simulink model "MADA3"  (R2020a)
settings: Solver=ode4  StartTime=start_time  StopTime=stop_time  FixedStep=fixed_step_size  MaxStep=1e-4  RelTol=1e-3
undefined symbols (not defined in the file): J, Ki, Kp, Lr, Ls, M, p, Rr, Rs, T_23, T_32
settings Model: Creator=deric  LastModifiedBy=deric

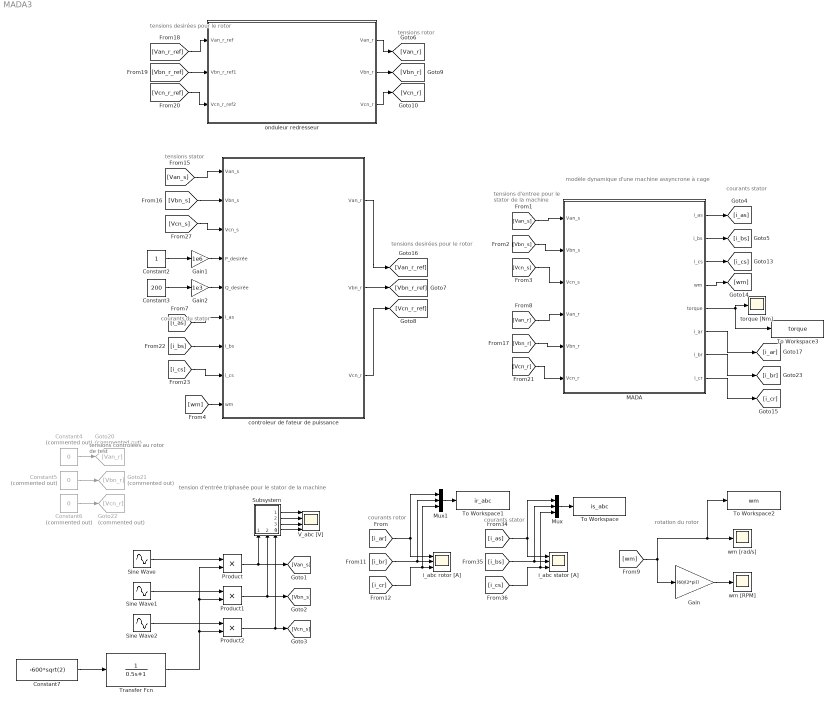
== system MADA3 ==
  note: tensions desirées
      | pour le rotor
  note: courants stator
  note: courants rotor
  note: tensions stator
  note: rotation du rotor
  note: tensions rotor
  note: tensions desirées
      | pour le rotor
  note: tensions controlées
      | au rotor de test
  note: tensions d'entree pour
      | le stator de la machine
  note: modèle dynamique d'une machine assyncrone à cage
  note: courants stator
  note: tension d'entrée triphasée pour le stator de la machine
  note: courants du stator
  Constant2 : Constant
  Constant3 : Constant  Value=200
  Constant4 : Constant  Commented=on  Value=0
  Constant5 : Constant  Commented=on  Value=0
  Constant6 : Constant  Commented=on  Value=0
  Constant7 : Constant  Value=-600*sqrt(2)
  Gain : Gain  Gain=(60/(2*pi))
  Gain1 : Gain  Gain=1e6
  Gain2 : Gain  Gain=1e3
  Goto20 : Goto  Commented=on  GotoTag=Van_r
  Goto21 : Goto  Commented=on  GotoTag=Vbn_r
  Goto22 : Goto  Commented=on  GotoTag=Vcn_r
  MADA : Subsystem
  Mux : Mux  Inputs=3
  Mux1 : Mux  Inputs=3
  Product : Product
  Product1 : Product
  Product2 : Product
  Sine Wave : Sin  Frequency=50*2*pi  SampleTime=0
  Sine Wave1 : Sin  Frequency=50*2*pi  Phase=-2*pi/3  SampleTime=0
  Sine Wave2 : Sin  Frequency=50*2*pi  Phase=(2*pi)/3  SampleTime=0
  Subsystem : Subsystem
      settings: PortSchema="{\"entries\":[{\"content\":{\"sides\":[{\"content\":{\"connectorIds\":[]},\"type\":\"ConnectorPlacement.EquallySpacedRectSide\",\"uuid\":\"f85b66a8-0283-4540-940c-33deb3ca5510\"},{\"content\":{\"connectorIds\":[\"Out1\",\"Out2\",\"Out3\",\"Out4\"],\"side\":\"RIGHT\"},\"type\":\"ConnectorPlacement.EquallySpacedRectSide\",\"uuid\":\"e99f7d2c-d092-4cab-bef3-1d0691980dab\"},{\"content\":{\"connectorIds\":[],\"side\":\"TOP\"},\"type\":\"ConnectorPlacement.EquallySpacedRectSide\",\"uuid\":\"dc5a25e5-8be2-48e2-ba29-fa1fa10bdc19\"},{\"content\":{\"connectorIds\":[\"In1\",\"In2\",\"In3\"],\"side\":\"BOTTOM\"},\"type\":\"ConnectorPlacement.EquallySpacedRectSide\",\"uuid\":\"6c390d1e-5fa5-44b0-aac6-b431b338384d\"}]},\"type\":\"ConnectorPlacement.EquallySpacedConnector\",\"uuid\":\"6ae22648-050b-430b-93b5-6047f057b4ba\"}],\"packageUris\":[\"http://schema.mathworks.com/mf0/Connector/19700101\"],\"version\":\"1.0\"}"
  To Workspace : ToWorkspace  VariableName=is_abc  SampleTime=-1
  To Workspace1 : ToWorkspace  VariableName=ir_abc  SampleTime=-1
  To Workspace2 : ToWorkspace  VariableName=wm  SampleTime=-1
  To Workspace3 : ToWorkspace  VariableName=torque  SampleTime=-1
  Transfer Fcn : TransferFcn  Denominator=[0.5 1]
  V_abc [V] : Scope  NumInputPorts=4
  controleur de fateur de puissance : Subsystem
  i_abc rotor [A] : Scope  NumInputPorts=3
  i_abc stator [A] : Scope  NumInputPorts=3
  onduleur redresseur : Subsystem
  torque [Nm] : Scope
  wm [RPM] : Scope
  wm [rad/s] : Scope
  wires:
  [wm] -> To Workspace2/1, wm [rad/s]/1, Gain/1
  Gain/1 -> wm [RPM]/1
  [Van_r_ref] -> onduleur redresseur/1(Van_r_ref)
  [Vbn_r_ref] -> onduleur redresseur/2(Vbn_r_ref1)
  [Vcn_r_ref] -> onduleur redresseur/3(Vcn_r_ref2)
  onduleur redresseur/1(Van_r) -> [Van_r]
  onduleur redresseur/2(Vbn_r) -> [Vbn_r]
  onduleur redresseur/3(Vcn_r) -> [Vcn_r]
  [i_ar] -> i_abc rotor [A]/1, Mux1/1
  [i_br] -> Mux1/2, i_abc rotor [A]/2
  [i_cr] -> Mux1/3, i_abc rotor [A]/3
  [i_cs] -> Mux/3, i_abc stator [A]/3
  [i_as] -> Mux/1, i_abc stator [A]/1
  [i_bs] -> Mux/2, i_abc stator [A]/2
  Mux/1 -> To Workspace/1
  Mux1/1 -> To Workspace1/1
  MADA/3(i_cs) -> [i_cs]
  MADA/4(wm) -> [wm]
  [Vcn_s] -> MADA/3(Vcn_s)
  [Van_s] -> MADA/1(Van_s)
  MADA/5(torque) -> To Workspace3/1, torque [Nm]/1
  [Vbn_s] -> MADA/2(Vbn_s)
  MADA/1(i_as) -> [i_as]
  MADA/2(i_bs) -> [i_bs]
  Subsystem/3(Out3) -> V_abc [V]/3
  Subsystem/2(Out2) -> V_abc [V]/2
  Subsystem/1(Out1) -> V_abc [V]/1
  Subsystem/4(Out4) -> V_abc [V]/4
  [Van_r] -> MADA/4(Van_r)
  [Vbn_r] -> MADA/5(Vbn_r)
  [Vcn_r] -> MADA/6(Vcn_r)
  Constant2/1 -> Gain1/1
  Constant3/1 -> Gain2/1
  Constant6/1 -> Goto22/1
  Constant5/1 -> Goto21/1
  Constant4/1 -> Goto20/1
  MADA/6(i_ar) -> [i_ar]
  MADA/7(i_br) -> [i_br]
  MADA/8(i_cr) -> [i_cr]
  Sine Wave/1 -> Product/1
  Sine Wave1/1 -> Product1/1
  Sine Wave2/1 -> Product2/1
  Product/1 -> Subsystem/1(In1), [Van_s]
  Product1/1 -> Subsystem/2(In2), [Vbn_s]
  Product2/1 -> Subsystem/3(In3), [Vcn_s]
  Constant7/1 -> Transfer Fcn/1
  Transfer Fcn/1 -> Product2/2, Product1/2, Product/2
  controleur de fateur de puissance/1(Van_r) -> [Van_r_ref]
  controleur de fateur de puissance/2(Vbn_r) -> [Vbn_r_ref]
  controleur de fateur de puissance/3(Vcn_r) -> [Vcn_r_ref]
  Gain1/1 -> controleur de fateur de puissance/4(P_desirée)
  Gain2/1 -> controleur de fateur de puissance/5(Q_desirée)
  [Vbn_s] -> controleur de fateur de puissance/2(Vbn_s)
  [Van_s] -> controleur de fateur de puissance/1(Van_s)
  [Vcn_s] -> controleur de fateur de puissance/3(Vcn_s)
  [i_as] -> controleur de fateur de puissance/6(i_as)
  [i_bs] -> controleur de fateur de puissance/7(i_bs)
  [i_cs] -> controleur de fateur de puissance/8(i_cs)
  [wm] -> controleur de fateur de puissance/9(wm)

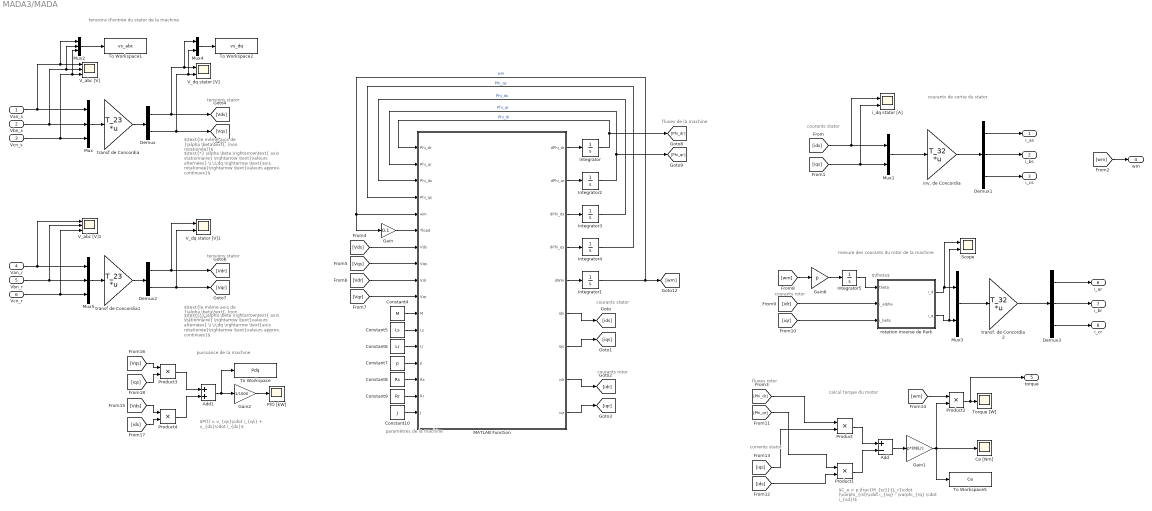
== system MADA3/MADA ==
  note: $\text{*} \alpha \beta \rightarrow\text{ axis stationnaire} \rightarrow \text{valeurs alternées} \\ \;\;dq \rightarrow \text{axis rotationée}\rightarrow \text{valeurs approx. continues}$
  note: $\text{le même axis de }\alpha \beta\text{, (non rotationée)}$
  note: paramètres de
      | la machine
  note: tensions stator
  note: courants stator
  note: currents stator
  note: fluxes rotor
  note: courants rotor
  note: courants stator
  note: fluxes de la machine
  note: calcul torque du motor
  note: courants de sortie du stator
  note: tensions d'entrée du stator de la machine
  note: $C_e = p \frac{M_{sr}}{L_r}\cdot (\varphi_{rd}\cdot i_{sq} - \varphi_{rq} \cdot i_{sd})$
  note: $P(t) = v_{qs}\cdot i_{qs} + v_{ds}\cdot i_{ds}$
  note: puissance de la machine
  note: $\text{le même axis de }\alpha \beta\text{, (non rotationée)}$
  note: $\text{*} \alpha \beta \rightarrow\text{ axis stationnaire} \rightarrow \text{valeurs alternées} \\ \;\;dq \rightarrow \text{axis rotationée}\rightarrow \text{valeurs approx. continues}$
  note: tensions stator
  note: $\theta$
  note: courants rotor
  note: mesure des courants du rotor de la machine
  Van_s : Inport
  Vbn_s : Inport  Port=2
  Vcn_s : Inport  Port=3
  Van_r : Inport  Port=4
  Vbn_r : Inport  Port=5
  Vcn_r : Inport  Port=6
  Add : Sum  Inputs=+-
  Add1 : Sum
  Ce [Nm] : Scope
  Constant10 : Constant  Value=J
  Constant4 : Constant  Value=M
  Constant5 : Constant  Value=Ls
  Constant6 : Constant  Value=Lr
  Constant7 : Constant  Value=p
  Constant8 : Constant  Value=Rs
  Constant9 : Constant  Value=Rr
  Demux : Demux  Outputs=2
  Demux1 : Demux  Outputs=3
  Demux2 : Demux  Outputs=2
  Demux3 : Demux  Outputs=3
  Gain : Gain  Gain=0.1
  Gain1 : Gain  Gain=p*(M/Lr)
  Gain2 : Gain  Gain=1/1000
  Gain6 : Gain  Gain=p
  Integrator{,1..5} (6 alike) : Integrator
  MATLAB Function : MATLAB Function  TreatAsAtomicUnit=on
  Mux : Mux  Inputs=3
  Mux1 : Mux  Inputs=2
  Mux2 : Mux  Inputs=3
  Mux3 : Mux  Inputs=2
  Mux4 : Mux  Inputs=2
  Mux5 : Mux  Inputs=3
  P(t) [kW] : Scope
  Product{,1..4} (5 alike) : Product
  Scope : Scope  NumInputPorts=2
  To Workspace : ToWorkspace  VariableName=Pdq  SampleTime=-1
  To Workspace1 : ToWorkspace  VariableName=vs_abc  SampleTime=-1
  To Workspace2 : ToWorkspace  VariableName=vs_dq  SampleTime=-1
  To Workspace5 : ToWorkspace  VariableName=Ce  SampleTime=-1
  Torque [W] : Scope
  V_abc [V] : Scope  NumInputPorts=3
  V_abc [V]1 : Scope  NumInputPorts=3
  V_dq stator [V] : Scope  NumInputPorts=2
  V_dq stator [V]1 : Scope  NumInputPorts=2
  i_dq stator [A] : Scope  NumInputPorts=2
  inv. de Concordia : Gain  Gain=T_32  Multiplication=Matrix(K*u)
  rotation inverse de Park : MATLAB Function  TreatAsAtomicUnit=on
  transf de Concordia : Gain  Gain=T_23  Multiplication=Matrix(K*u)
  transf de Concordia1 : Gain  Gain=T_23  Multiplication=Matrix(K*u)
  transf. de Concordia 2 : Gain  Gain=T_32  Multiplication=Matrix(K*u)
  i_as : Outport
  i_bs : Outport  Port=2
  i_cs : Outport  Port=3
  wm : Outport  Port=4
  torque : Outport  Port=5
  i_ar : Outport  Port=6
  i_br : Outport  Port=7
  i_cr : Outport  Port=8
  wires:
  Constant4/1 -> MATLAB Function/11(M)
  [ids] -> i_dq stator [A]/1, Mux1/1
  Constant6/1 -> MATLAB Function/13(Lr)
  [Vdr] -> MATLAB Function/9(Vdr)
  Mux/1 -> transf de Concordia/1
  MATLAB Function/1(dPhi_dr) -> Integrator/1
  Gain/1 -> MATLAB Function/6(Tload)
  [Vqr] -> MATLAB Function/10(Vqr)
  Integrator1/1 -> [wm], MATLAB Function/5(wm), Gain/1  "wm"
  MATLAB Function/7(iqs) -> [iqs]
  Demux/2 -> [Vqs], Mux4/2, V_dq stator [V]/2
  Demux/1 -> Mux4/1, V_dq stator [V]/1, [Vds]
  Vbn_s/1 -> Mux2/2, V_abc [V]/2, Mux/2
  Constant10/1 -> MATLAB Function/17(J)
  [Vds] -> MATLAB Function/7(Vds)
  Integrator2/1 -> MATLAB Function/2(Phi_qr), [Phi_qr]  "Phi_qr"
  Demux1/3 -> i_cs/1
  MATLAB Function/9(iqr) -> [iqr]
  Demux1/1 -> i_as/1
  MATLAB Function/4(dPhi_qs) -> Integrator4/1
  Integrator4/1 -> MATLAB Function/4(Phi_qs)  "Phi_qs"
  Constant7/1 -> MATLAB Function/14(p)
  Demux1/2 -> i_bs/1
  [iqs] -> i_dq stator [A]/2, Mux1/2
  Constant8/1 -> MATLAB Function/15(Rs)
  MATLAB Function/6(ids) -> [ids]
  MATLAB Function/3(dPhi_ds) -> Integrator3/1
  transf de Concordia/1 -> Demux/1
  Integrator/1 -> [Phi_dr], MATLAB Function/1(Phi_dr)  "Phi_dr"
  inv. de Concordia/1 -> Demux1/1
  MATLAB Function/8(idr) -> [idr]
  MATLAB Function/5(dWm) -> Integrator1/1
  Constant5/1 -> MATLAB Function/12(Ls)
  Mux1/1 -> inv. de Concordia/1
  [Vqs] -> MATLAB Function/8(Vqs)
  Constant9/1 -> MATLAB Function/16(Rr)
  Integrator3/1 -> MATLAB Function/3(Phi_ds)  "Phi_ds"
  MATLAB Function/2(dPhi_qr) -> Integrator2/1
  Vcn_s/1 -> Mux2/3, V_abc [V]/3, Mux/3
  Van_s/1 -> Mux2/1, V_abc [V]/1, Mux/1
  [wm] -> wm/1
  [Phi_qr] -> Product1/1
  [ids] -> Product1/2
  Product/1 -> Add/1
  [Phi_dr] -> Product/1
  [iqs] -> Product/2
  Product1/1 -> Add/2
  Add/1 -> Gain1/1
  Gain1/1 -> To Workspace5/1, Product2/2, Ce [Nm]/1
  [wm] -> Product2/1
  Product2/1 -> torque/1, Torque [W]/1
  [Vqs] -> Product3/1
  [iqs] -> Product3/2
  [Vds] -> Product4/1
  [ids] -> Product4/2
  Product3/1 -> Add1/1
  Product4/1 -> Add1/2
  Gain2/1 -> P(t) [kW]/1
  Add1/1 -> To Workspace/1, Gain2/1
  Mux2/1 -> To Workspace1/1
  Mux4/1 -> To Workspace2/1
  Vcn_r/1 -> V_abc [V]1/3, Mux5/3
  Van_r/1 -> V_abc [V]1/1, Mux5/1
  transf de Concordia1/1 -> Demux2/1
  Demux2/1 -> V_dq stator [V]1/1, [Vdr]
  Demux2/2 -> [Vqr], V_dq stator [V]1/2
  Vbn_r/1 -> V_abc [V]1/2, Mux5/2
  Mux5/1 -> transf de Concordia1/1
  rotation inverse de Park/2(i_q) -> Scope/2, Mux3/2
  [wm] -> Gain6/1
  [idr] -> rotation inverse de Park/2(i_alpha)
  Demux3/1 -> i_ar/1
  Integrator5/1 -> rotation inverse de Park/1(theta)
  Demux3/2 -> i_br/1
  [iqr] -> rotation inverse de Park/3(i_beta)
  Gain6/1 -> Integrator5/1
  Mux3/1 -> transf. de Concordia 2/1
  transf. de Concordia 2/1 -> Demux3/1
  Demux3/3 -> i_cr/1
  rotation inverse de Park/1(i_d) -> Scope/1, Mux3/1

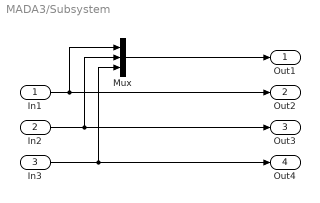
== system MADA3/Subsystem ==
  In1 : Inport
  In2 : Inport  Port=2
  In3 : Inport  Port=3
  Mux : Mux  Inputs=3
  Out1 : Outport
  Out2 : Outport  Port=2
  Out3 : Outport  Port=3
  Out4 : Outport  Port=4
  wires:
  In1/1 -> Mux/1, Out2/1
  In2/1 -> Out3/1, Mux/2
  In3/1 -> Mux/3, Out4/1
  Mux/1 -> Out1/1

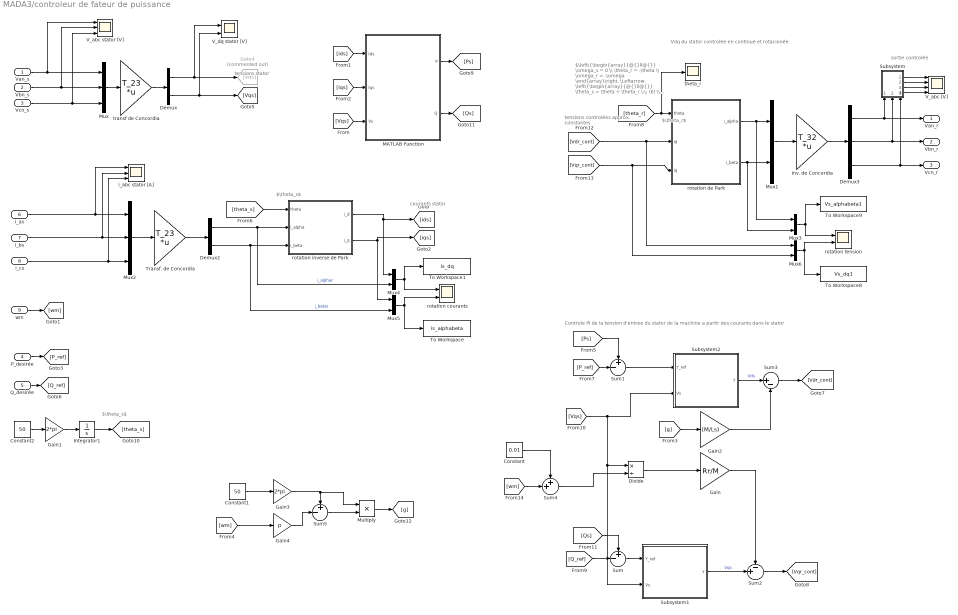
== system MADA3/controleur de fateur de puissance ==
  note: tensions stator
  note: courants stator
  note: $\theta_s$
  note: $\theta_s$
  note: Controle PI de la tension d'entree du stator de la machine a partir des courants dans le stator
  note: $\left\{\begin{array}{@{}ll@{}} \omega_s = 0 \\ \theta_r = -\theta \\ \omega_r = -\omega \end{array}\right. \Leftarrow \left\{\begin{array}{@{}ll@{}} \theta_s = \theta + \theta_r \;\; (6) \\ \omega_s = \omega + \omega_r \;\; (7) \\ \theta_s = 0 \;\;(17) \end{array}\right.$
  note: Vdq du stator controlée en continue et rotacionée
  note: tensions controlées
      | approx. constantes
  note: sortie controlée
  note: $\theta_r$
  Van_s : Inport
  Vbn_s : Inport  Port=2
  Vcn_s : Inport  Port=3
  P_desirée : Inport  Port=4
  Q_desirée : Inport  Port=5
  i_as : Inport  Port=6
  i_bs : Inport  Port=7
  i_cs : Inport  Port=8
  wm : Inport  Port=9
  Constant : Constant  Value=0.01
  Constant1 : Constant  Value=50
  Constant2 : Constant  Value=50
  Demux : Demux  Outputs=2
  Demux2 : Demux  Outputs=2
  Demux3 : Demux  Outputs=3
  Divide : Product  Inputs=*/
  Gain : Gain  Gain=Rr/M
  Gain1 : Gain  Gain=2*pi
  Gain2 : Gain  Gain=(M/Ls)
  Gain3 : Gain  Gain=2*pi
  Gain4 : Gain  Gain=p
  Goto4 : Goto  Commented=on  GotoTag=Vds
  Integrator1 : Integrator
  Inv. de Concordia : Gain  Gain=T_32  Multiplication=Matrix(K*u)
  MATLAB Function : MATLAB Function  TreatAsAtomicUnit=on
  Multiply : Product  Inputs=**
  Mux : Mux  Inputs=3
  Mux{1,3..6} (5 alike) : Mux  Inputs=2
  Mux2 : Mux  Inputs=3
  Subsystem : Subsystem
      settings: PortSchema="{\"entries\":[{\"content\":{\"sides\":[{\"content\":{\"connectorIds\":[]},\"type\":\"ConnectorPlacement.EquallySpacedRectSide\",\"uuid\":\"f85b66a8-0283-4540-940c-33deb3ca5510\"},{\"content\":{\"connectorIds\":[\"Out1\",\"Out2\",\"Out3\",\"Out4\"],\"side\":\"RIGHT\"},\"type\":\"ConnectorPlacement.EquallySpacedRectSide\",\"uuid\":\"e99f7d2c-d092-4cab-bef3-1d0691980dab\"},{\"content\":{\"connectorIds\":[],\"side\":\"TOP\"},\"type\":\"ConnectorPlacement.EquallySpacedRectSide\",\"uuid\":\"dc5a25e5-8be2-48e2-ba29-fa1fa10bdc19\"},{\"content\":{\"connectorIds\":[\"In1\",\"In2\",\"In3\"],\"side\":\"BOTTOM\"},\"type\":\"ConnectorPlacement.EquallySpacedRectSide\",\"uuid\":\"6c390d1e-5fa5-44b0-aac6-b431b338384d\"}]},\"type\":\"ConnectorPlacement.EquallySpacedConnector\",\"uuid\":\"6ae22648-050b-430b-93b5-6047f057b4ba\"}],\"packageUris\":[\"http://schema.mathworks.com/mf0/Connector/19700101\"],\"version\":\"1.0\"}"
  Subsystem1 : Subsystem
  Subsystem2 : Subsystem
  Sum : Sum  Inputs=+-|
  Sum1 : Sum  Inputs=+-|
  Sum2 : Sum  Inputs=-+|
  Sum3 : Sum  Inputs=|+-
  Sum4 : Sum  Inputs=++|
  Sum5 : Sum  Inputs=+-|
  To Workspace : ToWorkspace  VariableName=is_alphabeta  SampleTime=-1
  To Workspace1 : ToWorkspace  VariableName=is_dq  SampleTime=-1
  To Workspace8 : ToWorkspace  VariableName=Vs_dq1  SampleTime=-1
  To Workspace9 : ToWorkspace  VariableName=Vs_alphabeta1  SampleTime=-1
  Transf. de Concordia : Gain  Gain=T_23  Multiplication=Matrix(K*u)
  V_abc [V] : Scope  NumInputPorts=4
  V_abc stator [V] : Scope  NumInputPorts=3
  V_dq stator [V] : Scope  NumInputPorts=2
  i_abc stator [A] : Scope  NumInputPorts=3
  "rotation courants " : Scope  NumInputPorts=2
  rotation de Park : MATLAB Function  TreatAsAtomicUnit=on
  rotation inverse de Park : MATLAB Function  TreatAsAtomicUnit=on
  rotation tension : Scope  NumInputPorts=2
  theta_r : Scope
  transf de Concordia : Gain  Gain=T_23  Multiplication=Matrix(K*u)
  Van_r : Outport
  Vbn_r : Outport  Port=2
  Vcn_r : Outport  Port=3
  wires:
  transf de Concordia/1 -> Demux/1
  Van_s/1 -> V_abc stator [V]/1, Mux/1
  Vcn_s/1 -> V_abc stator [V]/3, Mux/3
  Demux/1 -> V_dq stator [V]/1, Goto4/1
  Vbn_s/1 -> V_abc stator [V]/2, Mux/2
  Mux/1 -> transf de Concordia/1
  Demux/2 -> [Vqs], V_dq stator [V]/2
  P_desirée/1 -> [P_ref]
  Q_desirée/1 -> [Q_ref]
  rotation inverse de Park/2(i_q) -> Mux5/1, [iqs]
  i_cs/1 -> i_abc stator [A]/3, Mux2/3
  Mux2/1 -> Transf. de Concordia/1
  i_as/1 -> i_abc stator [A]/1, Mux2/1
  rotation inverse de Park/1(i_d) -> Mux4/1, [ids]
  Transf. de Concordia/1 -> Demux2/1
  Demux2/1 -> Mux4/2, rotation inverse de Park/2(i_alpha)  "i_alphar"
  Mux5/1 -> To Workspace/1, "rotation courants "/2
  [theta_s] -> rotation inverse de Park/1(theta)
  i_bs/1 -> i_abc stator [A]/2, Mux2/2
  Mux4/1 -> To Workspace1/1, "rotation courants "/1
  Demux2/2 -> Mux5/2, rotation inverse de Park/3(i_beta)  "i_betar"
  Gain1/1 -> Integrator1/1
  Constant2/1 -> Gain1/1
  Sum/1 -> Subsystem1/1(Y_ref)
  [Q_ref] -> Sum/2
  Sum1/1 -> Subsystem2/1(Y_ref)
  [Ps] -> Sum1/1
  [P_ref] -> Sum1/2
  [Qs] -> Sum/1
  Subsystem/3(Out3) -> V_abc [V]/3
  Subsystem/4(Out4) -> V_abc [V]/4
  Subsystem/2(Out2) -> V_abc [V]/2
  rotation de Park/1(i_alpha) -> Mux3/1, Mux1/1
  Mux6/1 -> To Workspace8/1, rotation tension/2
  Mux3/1 -> To Workspace9/1, rotation tension/1
  [Vqr_cont] -> Mux6/2, rotation de Park/3(iq)
  Inv. de Concordia/1 -> Demux3/1
  Mux1/1 -> Inv. de Concordia/1
  [Vdr_cont] -> Mux6/1, rotation de Park/2(id)
  Demux3/2 -> Subsystem/2(In2), Vbn_r/1
  Subsystem/1(Out1) -> V_abc [V]/1
  Demux3/3 -> Subsystem/3(In3), Vcn_r/1
  [theta_r] -> rotation de Park/1(theta), theta_r/1
  rotation de Park/2(i_beta) -> Mux3/2, Mux1/2
  Demux3/1 -> Subsystem/1(In1), Van_r/1
  Divide/1 -> Gain/1
  Subsystem1/1(Y) -> Sum2/2  "Vqs"
  Sum2/1 -> [Vqr_cont]
  Gain/1 -> Sum2/1
  Subsystem2/1(Y) -> Sum3/1  "Vds"
  Sum3/1 -> [Vdr_cont]
  Gain2/1 -> Sum3/2
  MATLAB Function/1(P) -> [Ps]
  MATLAB Function/2(Q) -> [Qs]
  Integrator1/1 -> [theta_s]
  [Vqs] -> MATLAB Function/3(Vs)
  [ids] -> MATLAB Function/1(Ids)
  [iqs] -> MATLAB Function/2(Iqs)
  [Vqs] -> Subsystem1/2(Vs), Divide/1, Subsystem2/2(Vs)
  [wm] -> Sum4/2
  Sum4/1 -> Divide/2
  Constant/1 -> Sum4/1
  wm/1 -> [wm]
  [wm] -> Gain4/1
  Constant1/1 -> Gain3/1
  Gain3/1 -> Multiply/1, Sum5/1
  Gain4/1 -> Sum5/2
  Sum5/1 -> Multiply/2
  Multiply/1 -> [g]
  [g] -> Gain2/1

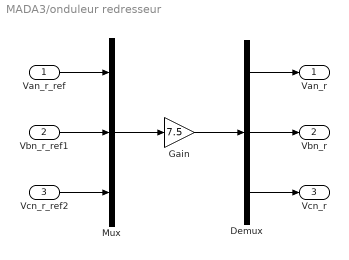
== system MADA3/onduleur redresseur ==
  Van_r_ref : Inport
  Vbn_r_ref1 : Inport  Port=2
  Vcn_r_ref2 : Inport  Port=3
  Demux : Demux  Outputs=3
  Gain : Gain  Gain=7.5
  Mux : Mux  Inputs=3
  Van_r : Outport
  Vbn_r : Outport  Port=2
  Vcn_r : Outport  Port=3
  wires:
  Mux/1 -> Gain/1
  Gain/1 -> Demux/1
  Van_r_ref/1 -> Mux/1
  Vbn_r_ref1/1 -> Mux/2
  Vcn_r_ref2/1 -> Mux/3
  Demux/1 -> Van_r/1
  Demux/2 -> Vbn_r/1
  Demux/3 -> Vcn_r/1

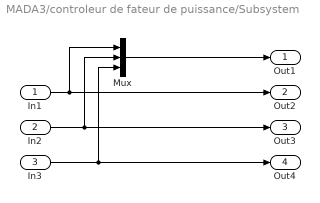
== system MADA3/controleur de fateur de puissance/Subsystem ==
  In1 : Inport
  In2 : Inport  Port=2
  In3 : Inport  Port=3
  Mux : Mux  Inputs=3
  Out1 : Outport
  Out2 : Outport  Port=2
  Out3 : Outport  Port=3
  Out4 : Outport  Port=4
  wires:
  In1/1 -> Mux/1, Out2/1
  In2/1 -> Out3/1, Mux/2
  In3/1 -> Mux/3, Out4/1
  Mux/1 -> Out1/1

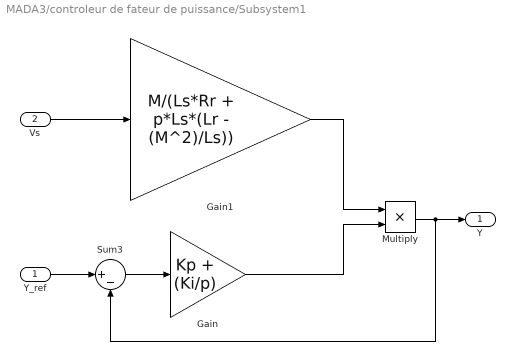
== system MADA3/controleur de fateur de puissance/Subsystem1 ==
  Y_ref : Inport
  Vs : Inport  Port=2
  Gain : Gain  Gain=Kp + (Ki/p)
  Gain1 : Gain  Gain=M/(Ls*Rr + p*Ls*(Lr - (M^2)/Ls))
  Multiply : Product  Inputs=**
  Sum3 : Sum  Inputs=|+-
  Y : Outport
  wires:
  Y_ref/1 -> Sum3/1
  Sum3/1 -> Gain/1
  Vs/1 -> Gain1/1
  Gain1/1 -> Multiply/1
  Gain/1 -> Multiply/2
  Multiply/1 -> Sum3/2, Y/1

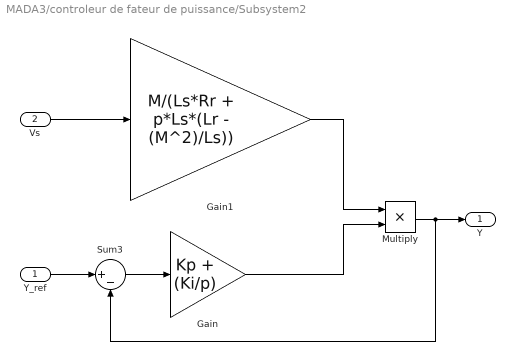
== system MADA3/controleur de fateur de puissance/Subsystem2 ==
  Y_ref : Inport
  Vs : Inport  Port=2
  Gain : Gain  Gain=Kp + (Ki/p)
  Gain1 : Gain  Gain=M/(Ls*Rr + p*Ls*(Lr - (M^2)/Ls))
  Multiply : Product  Inputs=**
  Sum3 : Sum  Inputs=|+-
  Y : Outport
  wires:
  Y_ref/1 -> Sum3/1
  Sum3/1 -> Gain/1
  Vs/1 -> Gain1/1
  Gain1/1 -> Multiply/1
  Gain/1 -> Multiply/2
  Multiply/1 -> Sum3/2, Y/1

== matlab function MADA3/MADA/rotation inverse de Park ==
  data: theta input; i_d output; i_alpha input; i_beta input; i_q output
function [i_d,i_q] = P_mtheta(theta, i_alpha, i_beta)
% P_theta Réalise la transformation inverse de Park.
%
% Cette fonction applique la transformation inverse de Park pour convertir les courants
% de l'axe alpha-bêta vers l'axe d-q (direct-quadrature).
% La transformation de Park est couramment utilisée dans le contrôle des moteurs AC
% et les onduleurs de puissance.
%
% Arguments :
%   theta (float): L'angle de rotation en radians.
%   i_d (float): Composant du courant sur l'axe alpha. 
%   i_q (float): Composant du courant sur l'axe bêta. 
%
% Retour :
%   i_alpha (float): Composant du courant sur l'axe direct après transformation.
%   i_beta (float): Composant du courant sur l'axe en quadrature après transformation.


P_mtheta = [cos(theta) sin(theta); -sin(theta) cos(theta)];
i_alphabeta = [i_alpha, i_beta]';

i_dq = P_mtheta*i_alphabeta; 

i_d = i_dq(1);
i_q = i_dq(2);

== matlab function MADA3/controleur de fateur de puissance/rotation de Park ==
  data: theta input; i_alpha output; id input; iq input; i_beta output
function [i_alpha,i_beta] = P_theta(theta, id, iq)
% P_theta Réalise la transformation de Park.
%
% Cette fonction applique la transformation de Park pour convertir 
% les courants de l'axe d-q (direct-quadrature) vers l'axe alpha-bêta.
% La transformation de Park est couramment utilisée dans le contrôle des 
% moteurs AC et les onduleurs de puissance.
%
% Arguments :
%   theta (float): L'angle de rotation en radians.
%   id (float): Composant du courant sur l'axe direct.
%   iq (float): Composant du courant sur l'axe en quadrature.
%
% Retour :
%   i_alpha (float): Composant du courant sur l'axe alpha après transformation.
%   i_beta (float): Composant du courant sur l'axe bêta après transformation.

P_theta = [cos(theta) -sin(theta); sin(theta) cos(theta)];
i_dq = [id, iq]';

i_alphabeta = P_theta*i_dq; 

i_alpha = i_alphabeta(1);
i_beta = i_alphabeta(2);

== matlab function MADA3/controleur de fateur de puissance/MATLAB Function ==
  data: Ids input; Iqs input; P output; Vs input; Q output
function [P,Q]  = fcn(Ids,Iqs,Vs)

P = Vs*Iqs;

Q = Vs*Ids;

== matlab function MADA3/MADA/MATLAB Function ==
  data: dPhi_dr output; dPhi_qr output; Phi_dr input; dPhi_ds output; dPhi_qs output; dWm output; Phi_qr input; Phi_ds input; Phi_qs input; wm input; Tload input; Vds input; Vqs input; Vdr input; Vqr input; M input; Ls input; Lr input; p input; ids output; iqs output; idr output; iqr output; Rs input; Rr input; J input
 function [dPhi_dr,dPhi_qr,dPhi_ds,dPhi_qs,dWm,ids,iqs,idr,iqr] = dynamique_machine(Phi_dr,Phi_qr,Phi_ds,Phi_qs,wm,Tload,Vds,Vqs,Vdr,Vqr,M,Ls,Lr,p,Rs,Rr,J)

% dPhi Calcul de la dérivée du flux de liaison magnétique, de la dérivée de la vitesse mécanique de l'arbre et du courant dans une machine asynchrone
% 
% Inputs:
%   Phis  : Vecteur des flux de liaison magnétiques
%   wm    : Vitesse mécanique de l'arbre
%   V     : Vecteur des tensions 
%   Tload : Couple de charge
%   ML    : Matrice d'inductance de la machine
%   p     : Nombre de pôles de la machine
%   R     : Matrice de résistance diagonale pour les enroulements stator et rotor
%
% Outputs:
%   dPhis : Vecteur de la dérivée du flux de liaison magnétique
%   dWm   : Dérivée de la vitesse mécanique de l'arbre
%   I     : Vecteur des courants 

% Initialisation de la vitesse angulaire statorique 
%à zéro (référentiel tournant)
ws = 0;

% Calcul de la vitesse angulaire rotorique à partir 
%de la vitesse mécanique
wr = -p*wm; % wm = W mécanique

% Calcul des courants à partir des flux de liaison magnétiques 
%et de la matrice d'inductance 
Phis = [Phi_ds,Phi_qs,Phi_dr,Phi_qr];
ML = [Ls 0 M 0; 0 Ls 0 M; M 0 Lr 0; 0 M 0 Lr];
LM=inv(ML);

I=LM*Phis';

ids=I(1);
iqs=I(2);
idr=I(3);
iqr=I(4);


% Calcul de la dérivée des flux de liaison magnétiques 
dPhi_ds = Vds - Rs*ids + ws*Phi_qs;
dPhi_qs = Vqs - Rs*iqs - ws*Phi_ds;
dPhi_dr = Vdr - Rr*idr + wr*Phi_qr;
dPhi_qr = Vqr - Rr*iqr - wr*Phi_dr;

% calcule le couple électromagnétique
%Tem = p*(Phi_ds*iqs - Phi_qs*ids);
Tem = p*(M/Lr)*(Phi_dr*iqs - Phi_qr*ids);

% Calcul de la dérivée de la vitesse mécanique
dWm = (1/J)*(Tem - Tload);

== matlab function MADA3/controleur de fateur de puissance/rotation inverse de Park ==
  data: theta input; i_d output; i_alpha input; i_beta input; i_q output
function [i_d,i_q] = P_mtheta(theta, i_alpha, i_beta)
% P_theta Réalise la transformation inverse de Park.
%
% Cette fonction applique la transformation inverse de Park pour convertir les courants
% de l'axe alpha-bêta vers l'axe d-q (direct-quadrature).
% La transformation de Park est couramment utilisée dans le contrôle des moteurs AC
% et les onduleurs de puissance.
%
% Arguments :
%   theta (float): L'angle de rotation en radians.
%   i_d (float): Composant du courant sur l'axe alpha. 
%   i_q (float): Composant du courant sur l'axe bêta. 
%
% Retour :
%   i_alpha (float): Composant du courant sur l'axe direct après transformation.
%   i_beta (float): Composant du courant sur l'axe en quadrature après transformation.


P_mtheta = [cos(theta) sin(theta); -sin(theta) cos(theta)];
i_alphabeta = [i_alpha, i_beta]';

i_dq = P_mtheta*i_alphabeta; 

i_d = i_dq(1);
i_q = i_dq(2);
